simulink model "ANfis"  (R2024a)
settings: Solver=VariableStepAuto  StartTime=0.0  StopTime=200  RelTol=1e-3
libraries: fuzblock x1, slpidlib x1
settings Model: Creator=FALCON  LastModifiedBy=FALCON

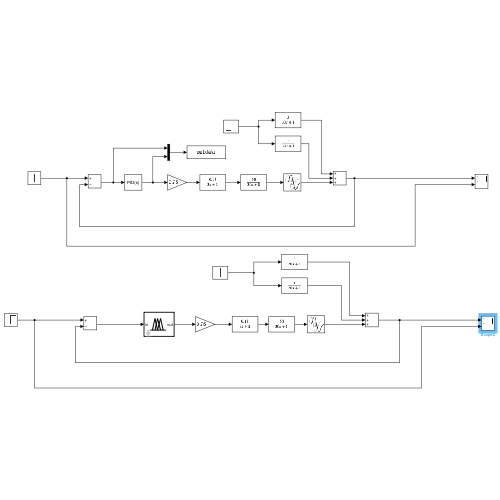
[thumbnail: Simulink's stored preview of the top-level diagram]
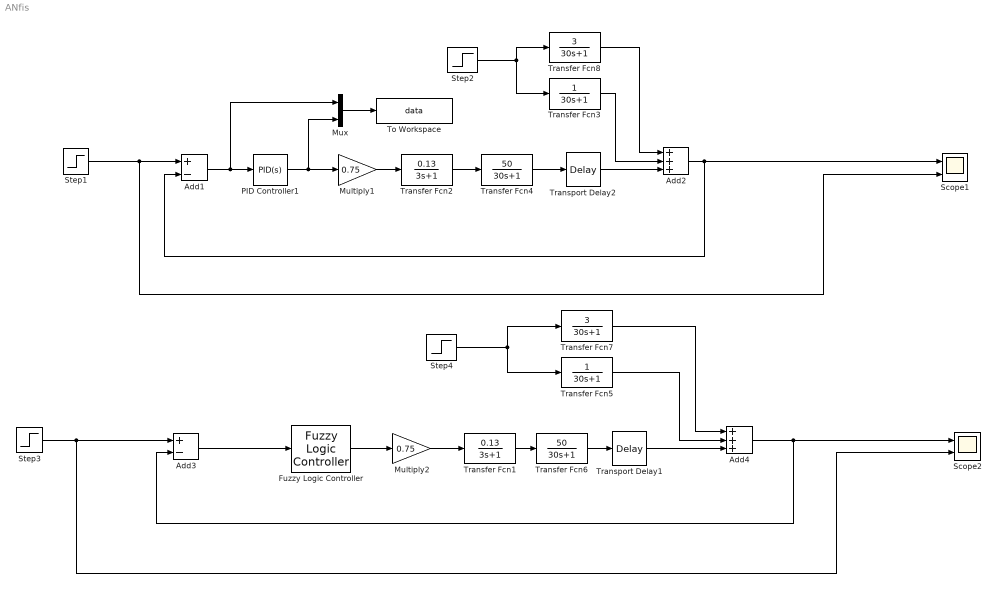
== system ANfis ==
  Add1 : Sum  Inputs=+-
  Add2 : Sum  Inputs=+++
  Add3 : Sum  Inputs=+-
  Add4 : Sum  Inputs=+++
  Fuzzy Logic Controller : fuzblock/Fuzzy Logic  Controller  FIS=aansif  OutputSampleNumber=101  DataType=double  FuzzifiedInputs=off  RuleFiringStrengths=off  RuleOutputs=off  AggregatedOutputs=off  SimulateUsing=Interpreted execution  OutOfRangeInputValueMessage=warning  NoRuleFiredMessage=warning  EmptyOutputFuzzySetMessage=warning
  Multiply1 : Gain  Gain=0.75
  Multiply2 : Gain  Gain=0.75
  Mux : Mux  Inputs=2
  PID Controller1 : slpidlib/PID Controller  Controller=PID  Form=Parallel  TimeDomain=Continuous-time  UseExternalTs=off  SampleTime=-1  IntegratorMethod=Forward Euler  FilterMethod=Forward Euler  ControllerParametersSource=internal  P=0.0341818015563616  I=0.00378271131176411  UseKiTs=off  D=-1.63079446969481  UseExternalDerivativeSource=off  N=0.0209602142952805  UseFilter=on  TunerSelectOption=Transfer Function Based (PID Tuner App)  InitialConditionSource=internal  InitialConditionForIntegrator=0  InitialConditionForFilter=0  DifferentiatorICPrevScaledInput=0  ExternalReset=none  TrackingMode=off  Kt=1  LimitOutput=off  SatLimitsSource=internal  UpperSaturationLimit=inf  LowerSaturationLimit=-inf  LinearizeAsGain=on  AntiWindupMode=none  Kb=1  LimitIntegrator=off  UpperIntegratorSaturationLimit=inf  LowerIntegratorSaturationLimit=-inf  POutMin=[]  POutMax=[]  IOutMin=[]  IOutMax=[]  DOutMin=[]  DOutMax=[]  NOutMin=[]  NOutMax=[]  SumOutMin=[]  SumOutMax=[]  SaturationOutMin=[]  SaturationOutMax=[]  PParamMin=[]  PParamMax=[]  IParamMin=[]  IParamMax=[]  DParamMin=[]  DParamMax=[]  NParamMin=[]  NParamMax=[]  KbParamMin=[]  KbParamMax=[]  KtParamMin=[]  KtParamMax=[]  KbOutMin=[]  KbOutMax=[]  KtOutMin=[]  KtOutMax=[]  IntegratorOutMin=[]  IntegratorOutMax=[]  FilterOutMin=[]  FilterOutMax=[]  SumI1OutMin=[]  SumI1OutMax=[]  SumI2OutMin=[]  SumI2OutMax=[]  SumI3OutMin=[]  SumI3OutMax=[]  SumI4OutMin=[]  SumI4OutMax=[]  SumDOutMin=[]  SumDOutMax=[]  DifferentiatorOutMin=[]  DifferentiatorOutMax=[]  FilterDiffOutCoefMin=[]  FilterDiffOutCoefMax=[]  ReciprocalOutMin=[]  ReciprocalOutMax=[]  SumDenOutMin=[]  SumDenOutMax=[]  SumNumOutMin=[]  SumNumOutMax=[]  DivideOutMin=[]  DivideOutMax=[]  UdiffTsProdOutMin=[]  UdiffTsProdOutMax=[]  NTsProdOutMin=[]  NTsProdOutMax=[]  UintegralTsProdOutMin=[]  UintegralTsProdOutMax=[]  UngainTsProdOutMin=[]  UngainTsProdOutMax=[]  ClampingZeroOutDataTypeStr=Inherit: Inherit via back propagation  ClampingZeroOutMin=[]  ClampingZeroOutMax=[]  FilterDenConstantOutDataTypeStr=Inherit: Inherit via back propagation  FilterDenConstantOutMin=[]  FilterDenConstantOutMax=[]  PCopyOutDataTypeStr=Inherit: Inherit via back propagation  PCopyOutMin=[]  PCopyOutMax=[]  NCopyOutDataTypeStr=Inherit: Inherit via back propagation  NCopyOutMin=[]  NCopyOutMax=[]  IntegratorContinuousStateAttributes=''  IntegratorStateMustResolveToSignalObject=off  IntegratorRTWStateStorageClass=Auto  FilterContinuousStateAttributes=''  FilterStateMustResolveToSignalObject=off  FilterRTWStateStorageClass=Auto  ParallelPVariant=InternalParameters  IdealPVariant=Disabled  IVariant=InternalParameters  DVariant=InternalParameters  IntegratorVariant=Continuous  SatVariant=Disabled  AWVariant=Passthrough  PCopyVariant=Disabled  TRVariant=Disabled  FdbkBlocksVariant=Forward  IdealPFdbkVariant=Disabled  SatFdbkVariant=Disabled  DerivativeFilterVariant=ContFilter  NVariant=InternalParameters  NCopyVariant=Disabled  FilterICVariant=InternalICsFilter  IntegratorICVariant=InternalICs  ExternalResetVariant=Disabled  TRSumVariant=Passthrough  SumFdbkVariant=Disabled  SumVariant=Sum_PID  TsampFilterVariant=InternalTs  TsampNgainVariant=Passthrough  TsampIntegralVariant=Disabled_SignalSpec  ExternalSaturationOutDataTypeStr=Inherit: Same as second input  DerivativeSourceVariant=ErrorSignal
  Scope1 : Scope  NumInputPorts=2
  Scope2 : Scope  NumInputPorts=2
  Step1 : Step  Time=0  SampleTime=0
  Step2 : Step  Time=0.01  After=0.01  SampleTime=0
  Step3 : Step  Time=0  SampleTime=0
  Step4 : Step  Time=0.01  After=0.01  SampleTime=0
  To Workspace : ToWorkspace  VariableName=data  SampleTime=-1
  Transfer Fcn1 : TransferFcn  Numerator=[0.13]  Denominator=[3 1]
  Transfer Fcn2 : TransferFcn  Numerator=[0.13]  Denominator=[3 1]
  Transfer Fcn3 : TransferFcn  Denominator=[30 1]
  Transfer Fcn4 : TransferFcn  Numerator=[50]  Denominator=[30 1]
  Transfer Fcn5 : TransferFcn  Denominator=[30 1]
  Transfer Fcn6 : TransferFcn  Numerator=[50]  Denominator=[30 1]
  Transfer Fcn7 : TransferFcn  Numerator=[3]  Denominator=[30 1]
  Transfer Fcn8 : TransferFcn  Numerator=[3]  Denominator=[30 1]
  Transport Delay1 : TransportDelay
  Transport Delay2 : TransportDelay
  wires:
  Transfer Fcn2/1 -> Transfer Fcn4/1
  Transfer Fcn4/1 -> Transport Delay2/1
  Step1/1 -> Add1/1, Scope1/2
  Add2/1 -> Add1/2, Scope1/1
  Multiply1/1 -> Transfer Fcn2/1
  Transport Delay2/1 -> Add2/3
  Step2/1 -> Transfer Fcn3/1, Transfer Fcn8/1
  Transfer Fcn3/1 -> Add2/2
  Transfer Fcn8/1 -> Add2/1
  Add1/1 -> Mux/1, PID Controller1/1
  PID Controller1/1 -> Mux/2, Multiply1/1
  Multiply2/1 -> Transfer Fcn1/1
  Add3/1 -> Fuzzy Logic Controller/1
  Transfer Fcn7/1 -> Add4/1
  Transfer Fcn5/1 -> Add4/2
  Add4/1 -> Add3/2, Scope2/1
  Transfer Fcn1/1 -> Transfer Fcn6/1
  Transfer Fcn6/1 -> Transport Delay1/1
  Step3/1 -> Scope2/2, Add3/1
  Transport Delay1/1 -> Add4/3
  Step4/1 -> Transfer Fcn7/1, Transfer Fcn5/1
  Fuzzy Logic Controller/1 -> Multiply2/1
  Mux/1 -> To Workspace/1
